simulink subsystem "FeedForwardAutoTune"  (R2023a)
settings: Solver=VariableStepAuto  StartTime=0.0  StopTime=10.0  RelTol=1e-3

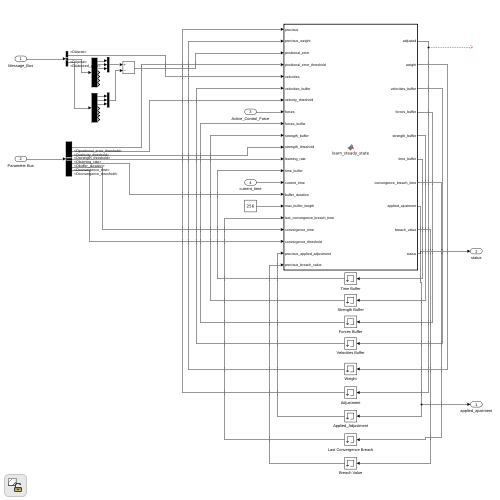
[thumbnail: Simulink's stored preview of the top-level diagram]
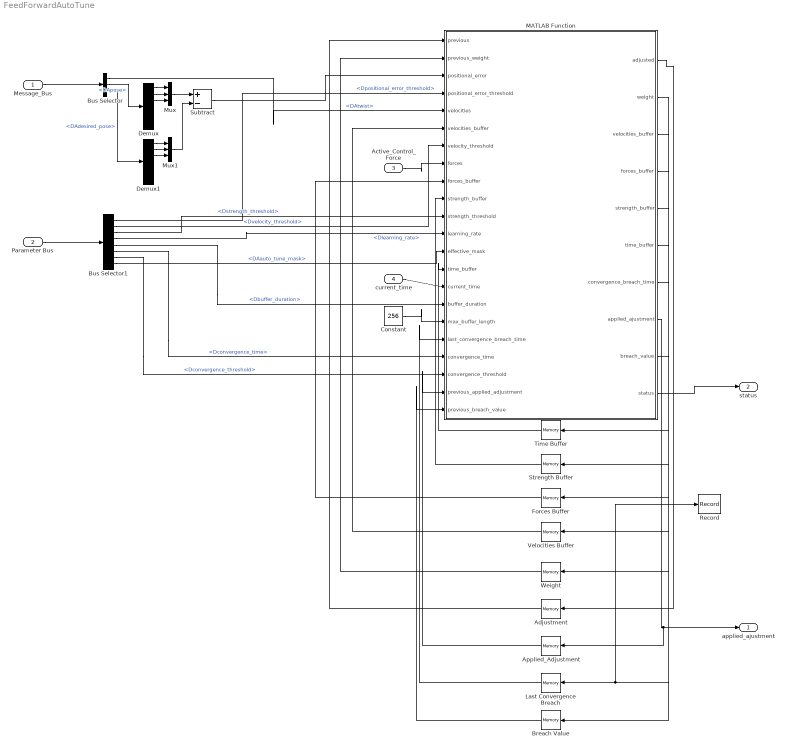
== system FeedForwardAutoTune ==
  Message_Bus : Inport
  Parameter Bus : Inport  Port=2
  Active_Control_Force : Inport  Port=3
  current_time : Inport  Port=4
  Adjustment : Memory  InitialCondition=[0;0;0;0;0;0]
  Applied_Adjustment : Memory  InitialCondition=[0;0;0;0;0;0]
  Breach Value : Memory  InitialCondition=[0;0;0;0;0;0]
  Bus Selector : BusSelector  OutputSignals=current_state.DAtwist,current_state.DApose,desired_pose.DAdesired_pose
  Bus Selector1 : BusSelector  OutputSignals=Dpositional_error_threshold,Dvelocity_threshold,Dstrength_threshold,Dlearning_rate,Dbuffer_duration,Dconvergence_time,Dconvergence_threshold,DAauto_tune_mask
  Constant : Constant  Value=256
  Demux : Demux  Outputs=7
  Demux1 : Demux  Outputs=7
  Forces Buffer : Memory  InitialCondition=zeros(6,256)
  Last Convergence Breach : Memory  InitialCondition=[0;0;0;0;0;0]
  MATLAB Function : MATLAB Function  TreatAsAtomicUnit=on
  Mux : Mux  Inputs=3
  Mux1 : Mux  Inputs=3
  Record : Record  FileSettingsInternal="{\"entries\":[{\"content\":{\"excelSettings\":{\"content\":{},\"type\":\"Streamout.ExcelSettings\"}},\"type\":\"Streamout.FileSettingStorage\",\"uuid\":\"\"}],\"packageUris\":[\"http:\\/\\/schema.mathworks.com\\/mf0\\/streamout_blocks\\/R2020a\"],\"version\":\"1.0\"}"  Layout=[1 1]  SignalsInternal="{\"entries\":[{\"content\":{\"signals\":[{\"content\":{\"blockPath\":[],\"dimensions\":[6,1],\"domain\":\"\",\"hasChildren\":true,\"lineColor\":\"#22b573\",\"port\":1,\"signalID\":8234,\"signalName\":\"MATLAB Function:7\"},\"type\":\"RecordBlkView.Signal\",\"uuid\":\"\"},{\"content\":{\"blockPath\":[],\"channel\":[1,1],\"dimensions\":[6,1],\"domain\":\"\",\"lineColor\":\"#0072bd\",\"parentID\":8234,\"port\":1,\"signalID\":8235,\"signalName\":\"MATLAB Function ...(+1263 chars)"  VisualizationBindings="{\"sparklinesplugin\":{\"info\":[{\"bindingParametersList\":[],\"subplotID\":1}]}}"
  Strength Buffer : Memory  InitialCondition=zeros(1, 256)
  Subtract : Sum  Inputs=+-
  Time Buffer : Memory  InitialCondition=zeros(1,256)
  Velocities Buffer : Memory  InitialCondition=zeros(6,256)
  Weight : Memory  InitialCondition=[0,0,0,0,0,0]
  applied_ajustment : Outport
  status : Outport  Port=2
  wires:
  Bus Selector/1 -> MATLAB Function/5(velocities)  "<DAtwist>"
  MATLAB Function/10(status) -> status/1
  Breach Value/1 -> MATLAB Function/22(previous_breach_value)
  Applied_Adjustment/1 -> MATLAB Function/21(previous_applied_adjustment)
  MATLAB Function/9(breach_value) -> Breach Value/1
  Mux1/1 -> Subtract/2
  Forces Buffer/1 -> MATLAB Function/9("forces_buffer ")
  MATLAB Function/3(velocities_buffer) -> Velocities Buffer/1
  Demux/1 -> Mux/1
  Demux/2 -> Mux/2
  Last Convergence Breach/1 -> MATLAB Function/18(last_convergence_breach_time)
  Bus Selector/2 -> Demux/1  "<DApose>"
  Time Buffer/1 -> MATLAB Function/14("time_buffer ")
  MATLAB Function/2(weight) -> Weight/1
  MATLAB Function/5(strength_buffer) -> Strength Buffer/1
  Demux1/3 -> Mux1/3
  Mux/1 -> Subtract/1
  Strength Buffer/1 -> MATLAB Function/10("strength_buffer ")
  Demux/3 -> Mux/3
  Message_Bus/1 -> Bus Selector/1
  Demux1/1 -> Mux1/1
  Weight/1 -> MATLAB Function/2(previous_weight)
  Demux1/2 -> Mux1/2
  MATLAB Function/8(applied_ajustment) -> applied_ajustment/1, Applied_Adjustment/1
  MATLAB Function/1(adjusted) -> Adjustment/1
  MATLAB Function/6(time_buffer) -> Time Buffer/1
  Velocities Buffer/1 -> MATLAB Function/6("velocities_buffer ")
  Adjustment/1 -> MATLAB Function/1(previous)
  MATLAB Function/4(forces_buffer) -> Forces Buffer/1
  Subtract/1 -> MATLAB Function/3(positional_error)
  Bus Selector/3 -> Demux1/1  "<DAdesired_pose>"
  Active_Control_Force/1 -> MATLAB Function/8(forces)
  current_time/1 -> MATLAB Function/15(current_time)
  Parameter Bus/1 -> Bus Selector1/1
  Bus Selector1/1 -> MATLAB Function/4(positional_error_threshold)  "<Dpositional_error_threshold>"
  Bus Selector1/2 -> MATLAB Function/7(velocity_threshold)  "<Dvelocity_threshold>"
  Bus Selector1/3 -> MATLAB Function/11(strength_threshold)  "<Dstrength_threshold>"
  Bus Selector1/4 -> MATLAB Function/12(learning_rate)  "<Dlearning_rate>"
  Bus Selector1/5 -> MATLAB Function/16(buffer_duration)  "<Dbuffer_duration>"
  Bus Selector1/6 -> MATLAB Function/19(convergence_time)  "<Dconvergence_time>"
  Bus Selector1/7 -> MATLAB Function/20(convergence_threshold)  "<Dconvergence_threshold>"
  Constant/1 -> MATLAB Function/17(max_buffer_length)
  Bus Selector1/8 -> MATLAB Function/13(effective_mask)  "<DAauto_tune_mask>"
  MATLAB Function/7(convergence_breach_time) -> Last Convergence Breach/1, Record/1

== matlab function FeedForwardAutoTune/MATLAB Function ==
function [adjusted, weight, velocities_buffer, forces_buffer, strength_buffer, time_buffer, convergence_breach_time, applied_ajustment, breach_value, status]   = learn_steady_state(previous, previous_weight, positional_error, positional_error_threshold, velocities, velocities_buffer, velocity_threshold, forces, forces_buffer, strength_buffer, strength_threshold, learning_rate, effective_mask, time_buffer, current_time, buffer_duration, max_buffer_length, last_convergence_breach_time, convergence_time, convergence_threshold, previous_applied_adjustment, previous_breach_value)

status = "Waiting";

%prevent nans
if(sum(isnan(previous)) ~= 0)
    previous = [0;0;0;0;0;0];
end

if(sum(isnan(previous_applied_adjustment)) ~= 0)
    previous_applied_adjustment = [0;0;0;0;0;0];
end

if(sum(isnan(previous_weight)) ~= 0)
    previous_weight = [1;1;1;1;1;1];
end

%pare buffer down to time
%find the max index which is within the time length
buffer_length = find(current_time - time_buffer > buffer_duration,1);
buffer_length = norm(buffer_length);

%enforce a max buffer length
buffer_length = min(max_buffer_length - 1, buffer_length) + 1;

%trim the buffer length
forces_buffer_temp = forces_buffer(:,1:buffer_length - 1);
strength_buffer_temp = strength_buffer(1:buffer_length - 1);
time_buffer_temp = time_buffer(1:buffer_length - 1);
velocities_buffer_temp = velocities_buffer(:,1:buffer_length - 1);

forces_buffer = zeros(6, 256);
forces_buffer(:, 2:buffer_length) = forces_buffer_temp;

strength_buffer = zeros(256,1);
strength_buffer(2:buffer_length) = strength_buffer_temp;

time_buffer = zeros(256,1);
time_buffer(2:buffer_length) = time_buffer_temp;
 
velocities_buffer = zeros(6, 256);
velocities_buffer(:, 2:buffer_length) = velocities_buffer_temp;

%append current time to buffer
time_buffer(1) = current_time;

%norm of absolute positional error
absolute_positional_error = norm(positional_error);

%only learn if velocity has been small for a while - ex hovering
absolute_velocities = norm(velocities(1:3));
if(absolute_velocities < velocity_threshold && absolute_positional_error < positional_error_threshold)

    %note status
    status = "Tracking";

    %strength of measrement determined by percentage of measurements being
    %under the velocity threshold
    strength_buffer(1) = 1;
    velocities_buffer(:, 1) = velocities;
    forces_buffer(:, 1) = forces;
    
    %only learn on strong measurements & measurements with a buffer length
    if(sum(strength_buffer) / buffer_length > strength_threshold)
        %if more force on average is being applied in a given direction,
        %increase the feed forward 
    
        %measured in newtons
        weight_step = abs(time_buffer(1) - time_buffer(2));
        weight = previous_weight + weight_step;
        adjusted = ((previous .* previous_weight + mean(forces_buffer,2) .* learning_rate .* weight_step)) ./ (previous_weight + learning_rate .* weight_step);
    else
        adjusted = previous;
        weight = previous_weight;
    end

else
    strength_buffer(1)  = 0;

    adjusted = previous;

    %append blank values for forces and previous velocities
    velocities_buffer(:,1) = [0;0;0;0;0;0];
    forces_buffer(:,1) = [0;0;0;0;0;0];
    weight = previous_weight;

end

applied_ajustment = previous_applied_adjustment;
convergence_breach_time = last_convergence_breach_time;
breach_value = previous_breach_value;

adjusted = adjusted .* effective_mask';

%determine the axis to apply leanring on 
target_axis = 1;
largest_magnitude = 0;
for i=1:6
    if(abs(adjusted(i)) > largest_magnitude)
        largest_magnitude = abs(adjusted(i));
        target_axis = i;
    end

    %check to see if the learning has convereged 
    if(abs(1 - adjusted(i) / previous_breach_value(i)) > convergence_threshold)
        convergence_breach_time(i) = current_time;
    
        %the value of adjsuted
        breach_value(i) = adjusted(i);
    end

end


%apply learning
if(current_time - convergence_breach_time(target_axis) > convergence_time && adjusted(target_axis) ~= 0)
    applied_ajustment(target_axis) = applied_ajustment(target_axis) + adjusted(target_axis);

    convergence_breach_time(target_axis) = current_time;

    %clear buffers
    weight = [0;0;0;0;0;0];
    disp("Here")

    strength_buffer = zeros(256,1);
    adjusted(target_axis) = 0;
end

%determine status
if(norm(effective_mask) == 0)
    status = "Disabled";
elseif(abs(1 - adjusted(i) / previous_breach_value(i)) > convergence_threshold * .1)
        status = "Converging";
end
